simulink model "Einfuehrung"  (R2014a)
settings: Solver=ode5  StartTime=0.0  StopTime=10.0  FixedStep=0.01  RelTol=1e-3
settings Model: Creator=s55812  LastModifiedBy=s55812

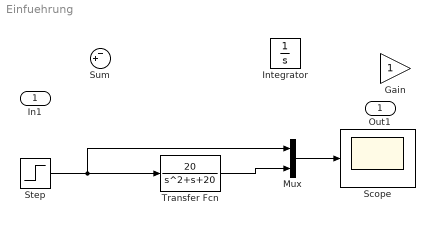
== system Einfuehrung ==
  In1 : Inport
  Gain : Gain
  Integrator : Integrator
  Mux : Mux  Inputs=2
  Scope : Scope
  Step : Step  SampleTime=0
  Sum : Sum  Inputs=-+|
  Transfer Fcn : TransferFcn  Numerator=[20]  Denominator=[1 1 20]
  Out1 : Outport
  wires:
  Step/1 -> Mux/1, Transfer Fcn/1
  Transfer Fcn/1 -> Mux/2
  Mux/1 -> Scope/1
